simulink model "SPWM Newscheme - Copy"  (R2019a)
settings: Solver=VariableStepAuto  StartTime=0.0  StopTime=10.0  RelTol=1e-3
libraries: powerlib x10
settings Model: Creator=simlab2020  LastModifiedBy=simlab2020

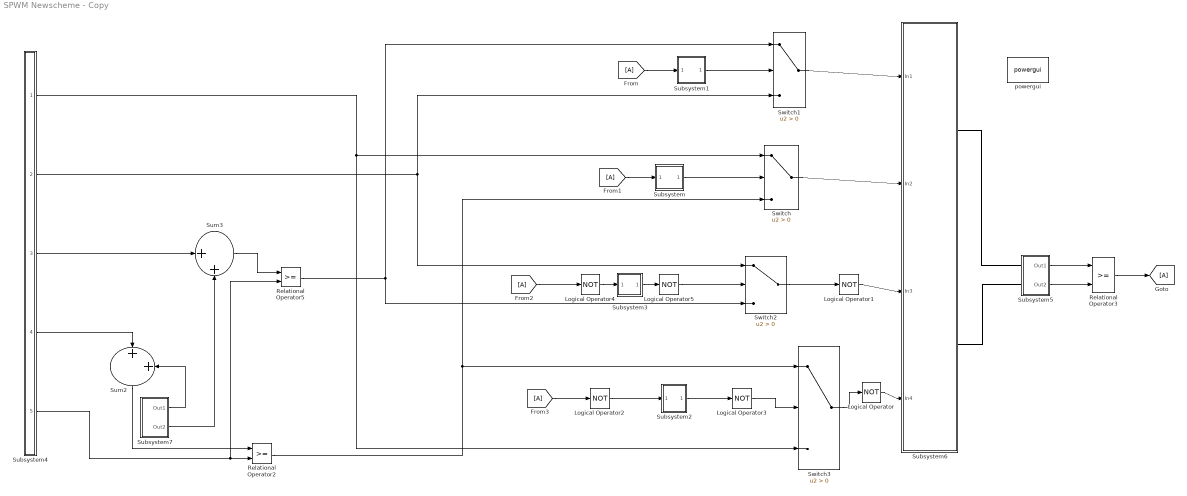
== system SPWM Newscheme - Copy ==
  Logical Operator{,1..5} (6 alike) : Logic  Operator=NOT  Inputs=1  AllPortsSameDT=off  OutDataTypeStr=boolean
  Relational Operator2 : RelationalOperator  OutDataTypeStr=boolean  RndMeth=Nearest
  Relational Operator3 : RelationalOperator  OutDataTypeStr=boolean  RndMeth=Nearest
  Relational Operator5 : RelationalOperator  OutDataTypeStr=boolean  RndMeth=Nearest
  Subsystem : Subsystem
  Subsystem1 : Subsystem
  Subsystem2 : Subsystem
  Subsystem3 : Subsystem
  Subsystem4 : Subsystem
  Subsystem5 : Subsystem
  Subsystem6 : Subsystem
  Subsystem7 : Subsystem
  Sum2 : Sum  Inputs=|++
  Sum3 : Sum  Inputs=|++
  Switch{,1..3} (4 alike) : Switch  Criteria=u2 > Threshold
  powergui : powerlib/powergui  Priority=1  SimulationMode=Continuous  SampleTime=50e-6  frequency=60  Iterations=50  frequencyindice=0  Pbase=100e6  ErrMax=1e-4  UnitsV=kV  UnitsW=MW  buscounter=0  FunctionMessages=off  echomessages=off  EnableUseOfTLC=off  CurrentSourceSwitches=on  DisableSnubberDevices=off  DisableRonSwitches=off  DisableVfSwitches=off  DisplayEquations=off  AutomaticDiscreteSolvers=off  SolverType=Tustin  Interpol=off  ExternalGateDelay=off  methode=off  Ts=0  x0status=blocks  SPID=off  SwTol=0  HookPort=off  NonlinearTolerance=0  nMaxIteration=15  ContinueOnMaxIteration=off  RestoreLinks=warning  ResistiveCurrentMeasurement=off  Frange=[0:2:500]  Ylog=off  Xlog=on  ShowGrid=off  save=off  variable=ZData  structure=current  ZoomFFT=off  StartTime=0.0  cycles=1  DisplayStyle=1  fundamental=50  FreqAxis=off  MaxFrequency=1000  frequencyindicesteady=1  RmsSteady=1  display=off
      settings: SourceProductName=Simscape Electrical
  wires:
  Subsystem7/2(Out2) -> Sum3/2
  Subsystem7/1(Out1) -> Sum2/2
  Relational Operator3/1 -> [A]
  [A] -> Logical Operator2/1
  [A] -> Logical Operator4/1
  Switch2/1 -> Logical Operator1/1
  Logical Operator3/1 -> Switch3/2
  Sum2/1 -> Relational Operator2/1
  Relational Operator5/1 -> Switch2/3, Switch1/1
  Subsystem2/1(Out1) -> Logical Operator3/1
  Subsystem3/1(Out1) -> Logical Operator5/1
  Logical Operator5/1 -> Switch2/2
  Subsystem1/1(Out1) -> Switch1/2
  Switch3/1 -> Logical Operator/1
  Subsystem/1(Out1) -> Switch/2
  Relational Operator2/1 -> Switch/3, Switch3/1
  Sum3/1 -> Relational Operator5/1
  Logical Operator2/1 -> Subsystem2/1(In1)
  [A] -> Subsystem/1(In1)
  Subsystem5/2(Out2) -> Relational Operator3/2
  Subsystem5/1(Out1) -> Relational Operator3/1
  Subsystem4/4(Out4) -> Sum2/1
  Subsystem4/5(Out5) -> Relational Operator2/2, Relational Operator5/2
  [A] -> Subsystem1/1(In1)
  Subsystem4/2(Out2) -> Switch2/1, Switch1/3
  Logical Operator/1 -> Subsystem6/4(In4)
  Switch/1 -> Subsystem6/2(In2)
  Switch1/1 -> Subsystem6/1(In1)
  Subsystem4/3(Out3) -> Sum3/1
  Logical Operator4/1 -> Subsystem3/1(In1)
  Subsystem4/1(Out1) -> Switch3/3, Switch/1
  Logical Operator1/1 -> Subsystem6/3(In3)
  connections:
  Subsystem6/RConn1 -- Subsystem5/LConn1
  Subsystem5/LConn2 -- Subsystem6/RConn2

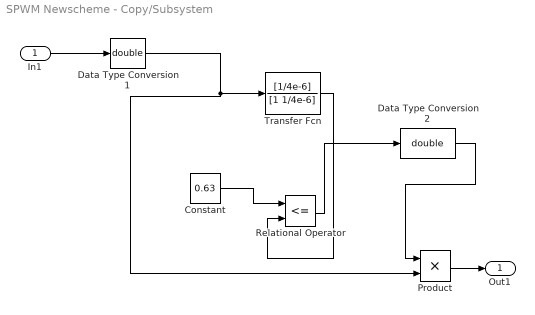
== system SPWM Newscheme - Copy/Subsystem ==
  In1 : Inport
  Constant : Constant  Value=0.63
  Data Type Conversion1 : DataTypeConversion  OutDataTypeStr=double
  Data Type Conversion2 : DataTypeConversion  OutDataTypeStr=double
  Product : Product
  Relational Operator : RelationalOperator  Operator=<=  OutDataTypeStr=boolean  RndMeth=Nearest
  Transfer Fcn : TransferFcn  Numerator=[1/4e-6]  Denominator=[1 1/4e-6]
  Out1 : Outport
  wires:
  In1/1 -> Data Type Conversion1/1
  Data Type Conversion1/1 -> Product/2, Transfer Fcn/1
  Transfer Fcn/1 -> Relational Operator/2
  Constant/1 -> Relational Operator/1
  Data Type Conversion2/1 -> Product/1
  Product/1 -> Out1/1
  Relational Operator/1 -> Data Type Conversion2/1

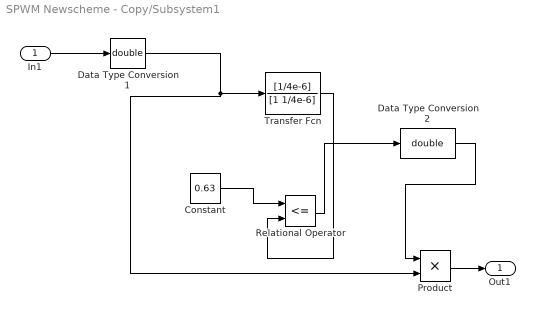
== system SPWM Newscheme - Copy/Subsystem1 ==
  In1 : Inport
  Constant : Constant  Value=0.63
  Data Type Conversion1 : DataTypeConversion  OutDataTypeStr=double
  Data Type Conversion2 : DataTypeConversion  OutDataTypeStr=double
  Product : Product
  Relational Operator : RelationalOperator  Operator=<=  OutDataTypeStr=boolean  RndMeth=Nearest
  Transfer Fcn : TransferFcn  Numerator=[1/4e-6]  Denominator=[1 1/4e-6]
  Out1 : Outport
  wires:
  In1/1 -> Data Type Conversion1/1
  Data Type Conversion1/1 -> Product/2, Transfer Fcn/1
  Transfer Fcn/1 -> Relational Operator/2
  Constant/1 -> Relational Operator/1
  Data Type Conversion2/1 -> Product/1
  Product/1 -> Out1/1
  Relational Operator/1 -> Data Type Conversion2/1

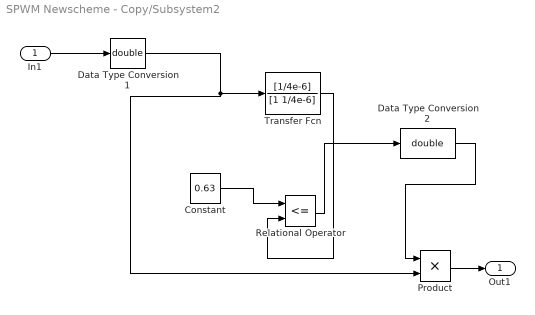
== system SPWM Newscheme - Copy/Subsystem2 ==
  In1 : Inport
  Constant : Constant  Value=0.63
  Data Type Conversion1 : DataTypeConversion  OutDataTypeStr=double
  Data Type Conversion2 : DataTypeConversion  OutDataTypeStr=double
  Product : Product
  Relational Operator : RelationalOperator  Operator=<=  OutDataTypeStr=boolean  RndMeth=Nearest
  Transfer Fcn : TransferFcn  Numerator=[1/4e-6]  Denominator=[1 1/4e-6]
  Out1 : Outport
  wires:
  In1/1 -> Data Type Conversion1/1
  Data Type Conversion1/1 -> Product/2, Transfer Fcn/1
  Transfer Fcn/1 -> Relational Operator/2
  Constant/1 -> Relational Operator/1
  Data Type Conversion2/1 -> Product/1
  Product/1 -> Out1/1
  Relational Operator/1 -> Data Type Conversion2/1

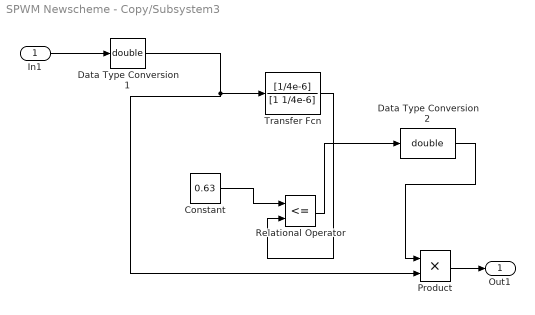
== system SPWM Newscheme - Copy/Subsystem3 ==
  In1 : Inport
  Constant : Constant  Value=0.63
  Data Type Conversion1 : DataTypeConversion  OutDataTypeStr=double
  Data Type Conversion2 : DataTypeConversion  OutDataTypeStr=double
  Product : Product
  Relational Operator : RelationalOperator  Operator=<=  OutDataTypeStr=boolean  RndMeth=Nearest
  Transfer Fcn : TransferFcn  Numerator=[1/4e-6]  Denominator=[1 1/4e-6]
  Out1 : Outport
  wires:
  In1/1 -> Data Type Conversion1/1
  Data Type Conversion1/1 -> Product/2, Transfer Fcn/1
  Transfer Fcn/1 -> Relational Operator/2
  Constant/1 -> Relational Operator/1
  Data Type Conversion2/1 -> Product/1
  Product/1 -> Out1/1
  Relational Operator/1 -> Data Type Conversion2/1

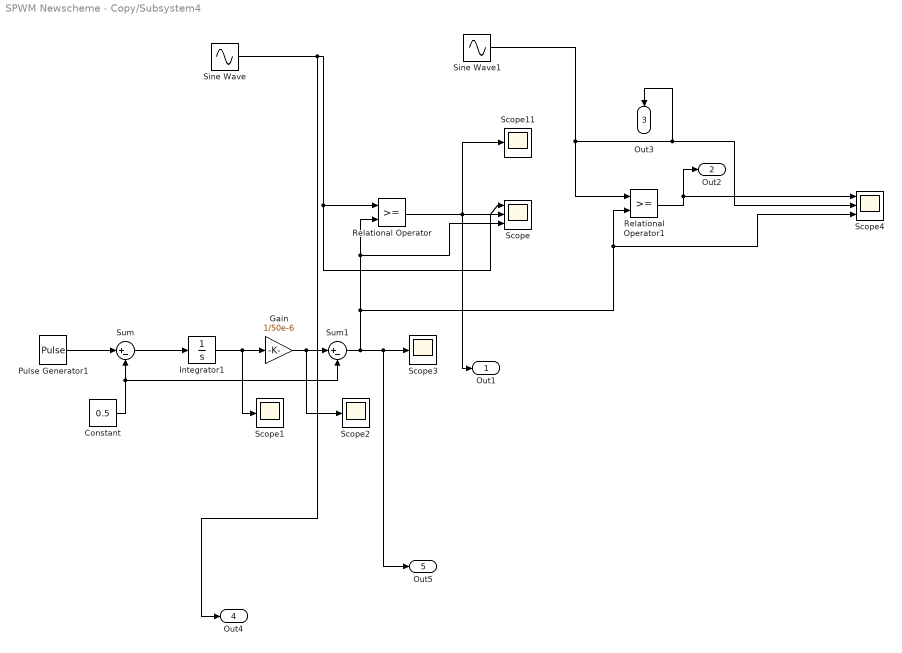
== system SPWM Newscheme - Copy/Subsystem4 ==
  Constant : Constant  Value=0.5
  Gain : Gain  Gain=1/50e-6
  Integrator1 : Integrator
  Pulse Generator1 : DiscretePulseGenerator  PulseType=Time based  Period=200e-6  PulseWidth=50
  Relational Operator : RelationalOperator  OutDataTypeStr=boolean  RndMeth=Nearest
  Relational Operator1 : RelationalOperator  OutDataTypeStr=boolean  RndMeth=Nearest
  Scope : Scope  NumInputPorts=3
  Scope{1..3,11} (4 alike) : Scope
  Scope4 : Scope  NumInputPorts=3
  Sine Wave : Sin  Amplitude=0.4  Frequency=2*pi*50  SampleTime=0
  Sine Wave1 : Sin  Amplitude=0.4  Frequency=2*pi*50  Phase=pi  SampleTime=0
  Sum : Sum  Inputs=|+-
  Sum1 : Sum  Inputs=|+-
  Out1 : Outport
  Out2 : Outport  Port=2
  Out3 : Outport  Port=3
  Out4 : Outport  Port=4
  Out5 : Outport  Port=5
  wires:
  Relational Operator1/1 -> Out2/1, Scope4/1
  Relational Operator/1 -> Out1/1, Scope11/1, Scope/1
  Integrator1/1 -> Scope1/1, Gain/1
  Gain/1 -> Scope2/1, Sum1/1
  Sum1/1 -> Out5/1, Scope3/1, Scope4/3, Relational Operator1/2, Scope/3, Relational Operator/2
  Pulse Generator1/1 -> Sum/1
  Sum/1 -> Integrator1/1
  Sine Wave1/1 -> Relational Operator1/1, Scope4/2, Out3/1
  Constant/1 -> Sum1/2, Sum/2
  Sine Wave/1 -> Out4/1, Scope/2, Relational Operator/1

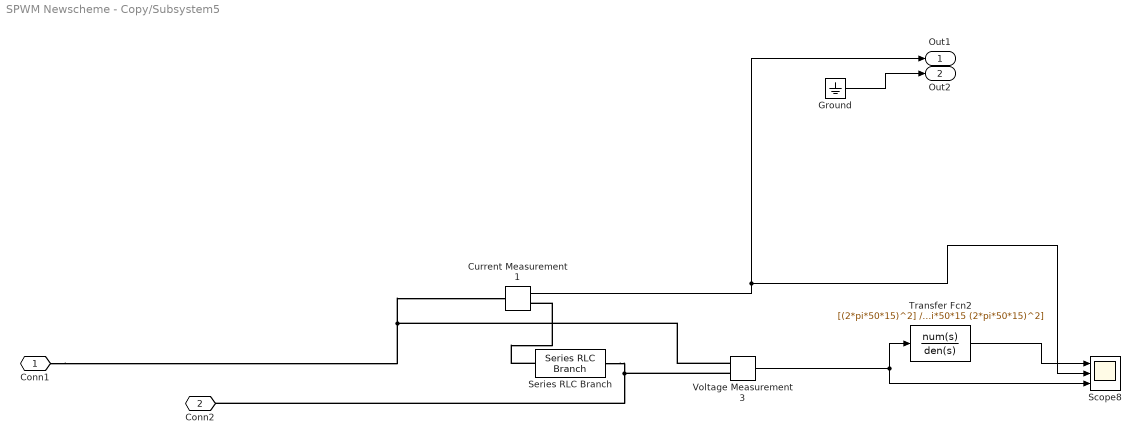
== system SPWM Newscheme - Copy/Subsystem5 ==
  Current Measurement1 : powerlib/Measurements/Current Measurement  PhasorSimulation=off  OutputType=Complex  PSBequivalent=0
      settings: SourceProductName=Simscape Electrical
  Ground : Ground
  Scope8 : Scope  NumInputPorts=3
  Series RLC Branch : powerlib/Elements/Series RLC Branch  LConnTagsString=__new0  RConnTagsString=__new0  BranchType=RL  Resistance=25  Inductance=225  SetiL0=off  InitialCurrent=0  Capacitance=0  Setx0=off  InitialVoltage=0  Measurements=None
      settings: SourceProductName=Simscape Electrical
  Transfer Fcn2 : TransferFcn  Numerator=[(2*pi*50*15)^2]  Denominator=[1 (1/0.707)*2*pi*50*15 (2*pi*50*15)^2]
  Voltage Measurement3 : powerlib/Measurements/Voltage Measurement  PhasorSimulation=off  OutputType=Complex  PSBequivalent=0
      settings: SourceProductName=Simscape Electrical
  Conn1 : PMIOPort  Side=Left
  Conn2 : PMIOPort  Port=2  Side=Left
  Out1 : Outport
  Out2 : Outport  Port=2
  wires:
  Voltage Measurement3/1 -> Transfer Fcn2/1, Scope8/3
  Current Measurement1/1 -> Out1/1, Scope8/2
  Transfer Fcn2/1 -> Scope8/1
  Ground/1 -> Out2/1
  connections:
  Series RLC Branch/LConn1 -- Current Measurement1/RConn1
  Voltage Measurement3/LConn1 -- Current Measurement1/LConn1 -- Conn1/RConn1
  Series RLC Branch/RConn1 -- Voltage Measurement3/LConn2 -- Conn2/RConn1

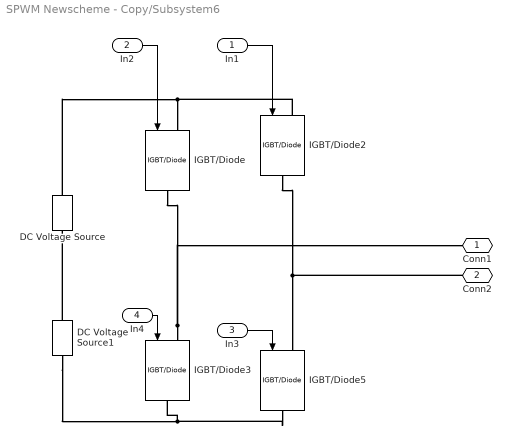
== system SPWM Newscheme - Copy/Subsystem6 ==
  In1 : Inport
  In2 : Inport  Port=2
  In3 : Inport  Port=3
  In4 : Inport  Port=4
  DC Voltage Source : powerlib/Electrical Sources/DC Voltage Source  Amplitude=165  Measurements=None
      settings: SourceProductName=Simscape Electrical
  DC Voltage Source1 : powerlib/Electrical Sources/DC Voltage Source  Amplitude=165  Measurements=None
      settings: SourceProductName=Simscape Electrical
  IGBT/Diode{,2..3,5} (4 alike) : powerlib/Power Electronics/IGBT//Diode  Ron=1e-3  Rs=1e5  Cs=47e-9  Measurements=off
      settings: SourceProductName=Simscape Electrical
  Conn1 : PMIOPort  Side=Right
  Conn2 : PMIOPort  Port=2  Side=Right
  wires:
  In2/1 -> IGBT/Diode/1
  In1/1 -> IGBT/Diode2/1
  In4/1 -> IGBT/Diode3/1
  In3/1 -> IGBT/Diode5/1
  connections:
  DC Voltage Source1/RConn1 -- DC Voltage Source/LConn1
  IGBT/Diode3/LConn1 -- IGBT/Diode/RConn1 -- Conn1/RConn1
  IGBT/Diode2/RConn1 -- IGBT/Diode5/LConn1 -- Conn2/RConn1
  DC Voltage Source/RConn1 -- IGBT/Diode2/LConn1 -- IGBT/Diode/LConn1
  DC Voltage Source1/LConn1 -- IGBT/Diode3/RConn1 -- IGBT/Diode5/RConn1

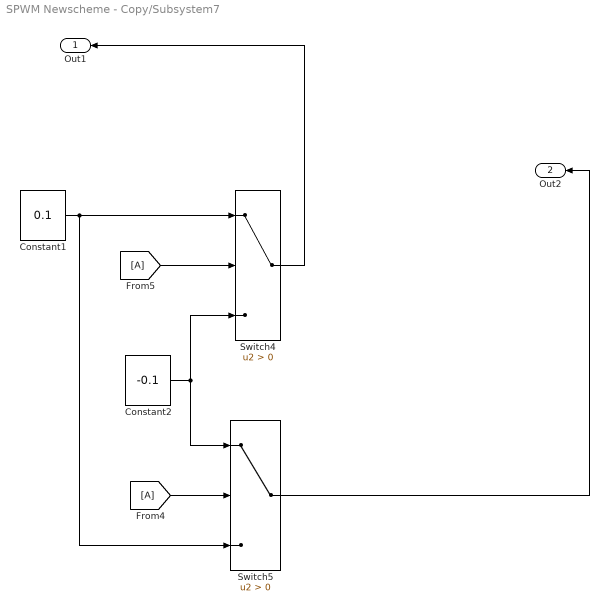
== system SPWM Newscheme - Copy/Subsystem7 ==
  Constant1 : Constant  Value=0.1
  Constant2 : Constant  Value=-0.1
  Switch4 : Switch  Criteria=u2 > Threshold
  Switch5 : Switch  Criteria=u2 > Threshold
  Out1 : Outport
  Out2 : Outport  Port=2
  wires:
  Constant2/1 -> Switch5/1, Switch4/3
  Constant1/1 -> Switch4/1, Switch5/3
  [A] -> Switch5/2
  [A] -> Switch4/2
  Switch5/1 -> Out2/1
  Switch4/1 -> Out1/1
